simulink model "Drone_Failure"  (R2020a)
settings: Solver=VariableStepAuto  StartTime=0.0  StopTime=10.0  RelTol=1e-3
undefined symbols (not defined in the file): b, desired_gamma, desired_phi, desired_theta, desired_X, desired_Y, desired_Z, g, Ir, Ixx, Iyy, Izz, k, l, m
libraries: simulink x3
settings Model: Creator=prans  LastModifiedBy=prans
settings SolverCC: MaxConsecutiveMinStep=5

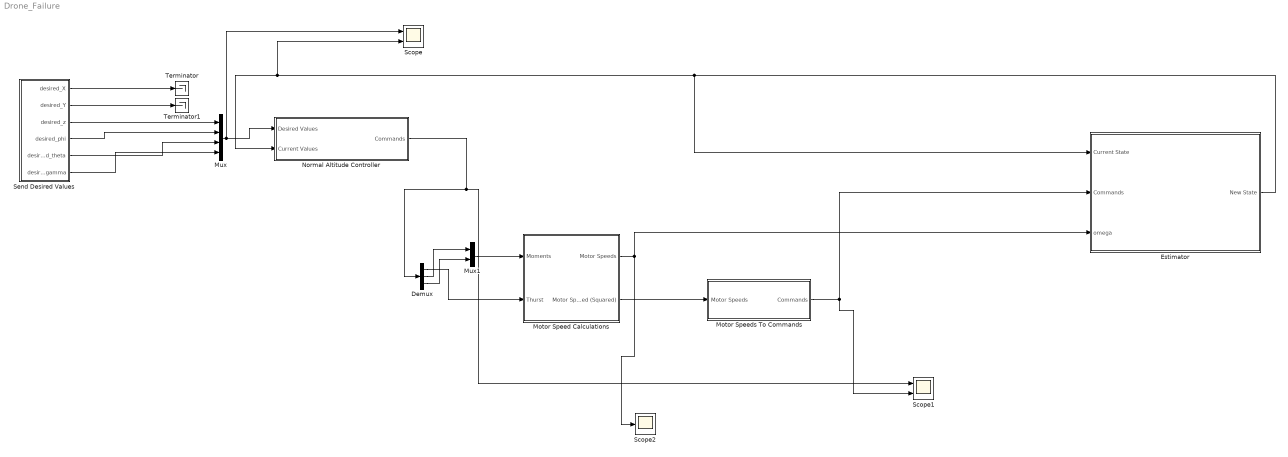
== system Drone_Failure ==
  Demux : Demux  Outputs=3
  Estimator : Subsystem
  Motor Speed Calculations : Subsystem
  Motor Speeds To Commands : Subsystem
  Mux : Mux
  Mux1 : Mux  Inputs=2
  Normal Altitude Controller : Subsystem
  Scope : Scope  NumInputPorts=2
  Scope1 : Scope  NumInputPorts=2
  Scope2 : Scope
  Send Desired Values : Subsystem
  Terminator : Terminator
  Terminator1 : Terminator
  wires:
  Send Desired Values/6(desired_gamma) -> Mux/4
  Send Desired Values/1(desired_X) -> Terminator/1
  Motor Speeds To Commands/1(Commands) -> Scope1/2, Estimator/2(Commands)
  Mux1/1 -> Motor Speed Calculations/1(Moments)
  Normal Altitude Controller/1(Commands) -> Scope1/1, Demux/1
  Motor Speed Calculations/1(Motor Speeds) -> Scope2/1, Estimator/3(omega)
  Send Desired Values/4(desired_phi) -> Mux/2
  Send Desired Values/5(desired_theta) -> Mux/3
  Demux/2 -> Mux1/1
  Send Desired Values/3(desired_z) -> Mux/1
  Send Desired Values/2(desired_Y) -> Terminator1/1
  Estimator/1(New State) -> Estimator/1(Current State), Scope/2, Normal Altitude Controller/2(Current Values)
  Demux/1 -> Motor Speed Calculations/2(Thurst)
  Mux/1 -> Scope/1, Normal Altitude Controller/1("Desired Values ")
  Demux/3 -> Mux1/2
  Motor Speed Calculations/2(Motor Speed (Squared)) -> Motor Speeds To Commands/1(Motor Speeds)

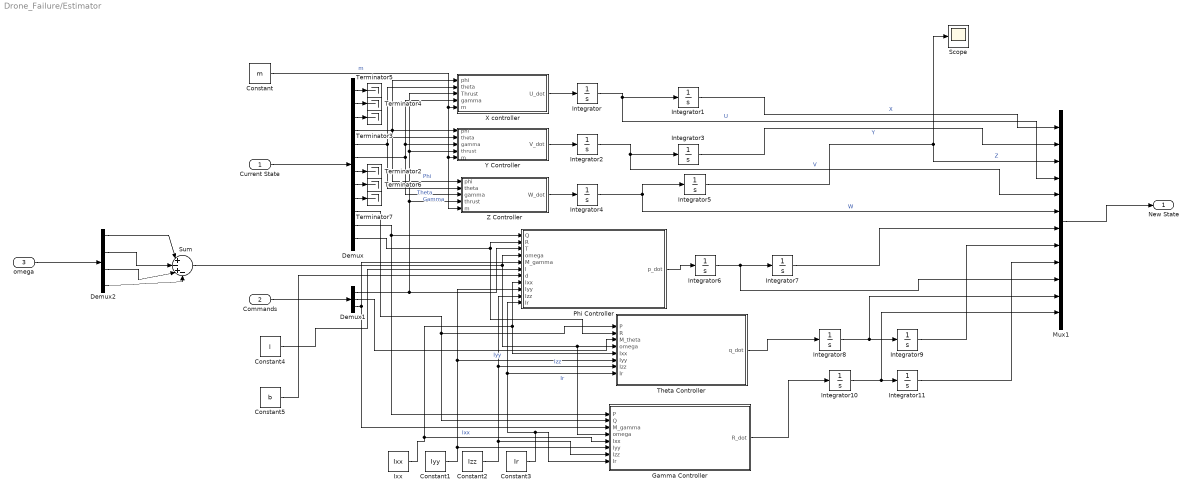
== system Drone_Failure/Estimator ==
  Current State : Inport
  Commands : Inport  Port=2
  omega : Inport  Port=3
  Constant : Constant  Value=m
  Constant1 : Constant  Value=Iyy
  Constant2 : Constant  Value=Izz
  Constant3 : Constant  Value=Ir
  Constant4 : Constant  Value=l
  Constant5 : Constant  Value=b
  Demux : Demux  Outputs=12
  Demux1 : Demux  Outputs=3
  Demux2 : Demux
  Gamma Controller : MATLAB Function  TreatAsAtomicUnit=on
  Integrator{,1..11} (12 alike) : Integrator
  Ixx : Constant  Value=Ixx
  Mux1 : Mux  Inputs=12
  Phi Controller : MATLAB Function  TreatAsAtomicUnit=on
  Scope : Scope
  Sum : Sum  Inputs=|+-+-
  Terminator{2..7} (6 alike) : Terminator
  Theta Controller : MATLAB Function  TreatAsAtomicUnit=on
  X controller : MATLAB Function  TreatAsAtomicUnit=on
  Y Controller : MATLAB Function  TreatAsAtomicUnit=on
  Z Controller : MATLAB Function  TreatAsAtomicUnit=on
  New State : Outport
  wires:
  Integrator8/1 -> Mux1/11, Integrator9/1
  Integrator6/1 -> Mux1/10, Integrator7/1
  Integrator9/1 -> Mux1/8
  Demux/11 -> Gamma Controller/1(P), Phi Controller/1(Q)
  Demux/9 -> Terminator7/1
  Demux/5 -> Y Controller/2(theta), X controller/2(theta), Z Controller/2(theta)  "Theta"
  Demux/2 -> Terminator4/1
  Demux/6 -> Y Controller/3(gamma), X controller/4(gamma), Z Controller/3(gamma)  "Gamma"
  Integrator1/1 -> Mux1/1  "X"
  Z Controller/1(W_dot) -> Integrator4/1
  Demux/3 -> Terminator3/1
  Gamma Controller/1(R_dot) -> Integrator10/1
  Current State/1 -> Demux/1
  Demux/10 -> Gamma Controller/2(Q), Theta Controller/1(P)
  Demux/8 -> Terminator6/1
  Demux/4 -> Z Controller/1(phi), Y Controller/1(phi), X controller/1(phi)  "Phi"
  Demux/7 -> Terminator2/1
  Integrator7/1 -> Mux1/7
  Demux/1 -> Terminator5/1
  Integrator11/1 -> Mux1/9
  Mux1/1 -> New State/1
  X controller/1(U_dot) -> Integrator/1
  Theta Controller/1(q_dot) -> Integrator8/1
  Integrator2/1 -> Integrator3/1, Mux1/5  "V"
  Phi Controller/1(p_dot) -> Integrator6/1
  Commands/1 -> Demux1/1
  Integrator3/1 -> Mux1/2  "Y"
  Y Controller/1(V_dot) -> Integrator2/1
  Demux/12 -> Theta Controller/2(R), Phi Controller/2(R)
  Integrator10/1 -> Mux1/12, Integrator11/1
  Integrator5/1 -> Scope/1, Mux1/3  "Z"
  Integrator/1 -> Integrator1/1, Mux1/4  "U"
  Integrator4/1 -> Integrator5/1, Mux1/6  "W"
  Ixx/1 -> Phi Controller/8(Ixx), Theta Controller/5(Ixx), Gamma Controller/5(Ixx)  "Ixx"
  Constant1/1 -> Phi Controller/9(Iyy), Theta Controller/6(Iyy), Gamma Controller/6(Iyy)  "Iyy"
  Constant2/1 -> Phi Controller/10(Izz), Theta Controller/7(Izz), Gamma Controller/7(Izz)  "Izz"
  Constant3/1 -> Phi Controller/11(Ir), Theta Controller/8(Ir), Gamma Controller/8(Ir)  "Ir"
  Constant/1 -> Z Controller/5(m), Y Controller/5(m), X controller/5(m)  "m"
  omega/1 -> Demux2/1
  Demux2/1 -> Sum/1
  Demux2/2 -> Sum/2
  Demux2/3 -> Sum/3
  Demux2/4 -> Sum/4
  Sum/1 -> Gamma Controller/4(omega), Theta Controller/4(omega), Phi Controller/4(omega)
  Demux1/1 -> X controller/3(Thrust), Y Controller/4(thrust), Z Controller/4(thrust), Phi Controller/3(T)
  Demux1/3 -> Phi Controller/5(M_gamma), Gamma Controller/3(M_gamma)
  Constant4/1 -> Phi Controller/6(l)
  Constant5/1 -> Phi Controller/7(d)
  Demux1/2 -> Theta Controller/3(M_theta)

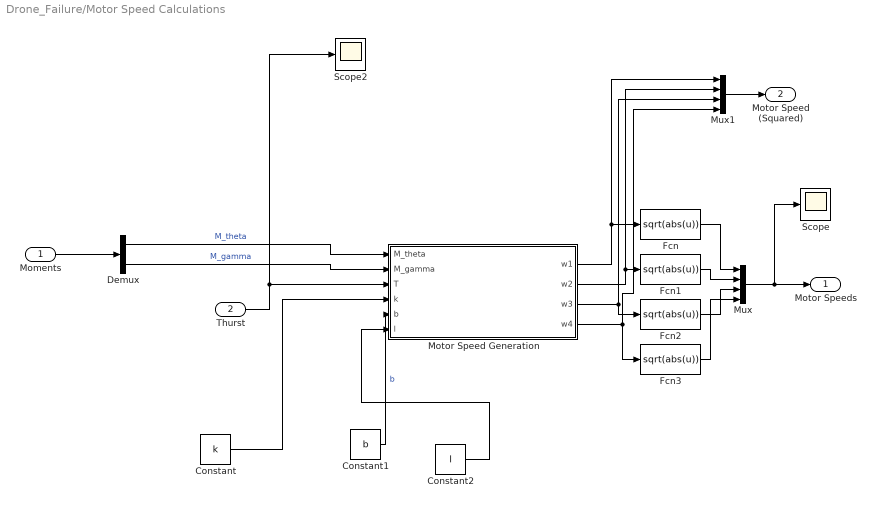
== system Drone_Failure/Motor Speed Calculations ==
  Moments : Inport
  Thurst : Inport  Port=2
  Constant : Constant  Value=k
  Constant1 : Constant  Value=b
  Constant2 : Constant  Value=l
  Demux : Demux  Outputs=2
  Fcn{,1..3} (4 alike) : Fcn  Expr=sqrt(abs(u))
  Motor Speed Generation : MATLAB Function  TreatAsAtomicUnit=on
  Mux : Mux
  Mux1 : Mux
  Scope : Scope
  Scope2 : Scope
  Motor Speeds : Outport
  Motor Speed (Squared) : Outport  Port=2
  wires:
  Motor Speed Generation/4(w4) -> Fcn3/1, Mux1/4
  Motor Speed Generation/2(w2) -> Mux1/2, Fcn1/1
  Thurst/1 -> Scope2/1, Motor Speed Generation/3(T)
  Motor Speed Generation/1(w1) -> Mux1/1, Fcn/1
  Motor Speed Generation/3(w3) -> Fcn2/1, Mux1/3
  Moments/1 -> Demux/1
  Mux/1 -> Scope/1, Motor Speeds/1
  Constant/1 -> Motor Speed Generation/4(k)
  Constant1/1 -> Motor Speed Generation/5(b)  "b"
  Demux/1 -> Motor Speed Generation/1(M_theta)  "M_theta"
  Demux/2 -> Motor Speed Generation/2(M_gamma)  "M_gamma"
  Constant2/1 -> Motor Speed Generation/6(l)
  Fcn/1 -> Mux/1
  Fcn1/1 -> Mux/2
  Fcn2/1 -> Mux/3
  Fcn3/1 -> Mux/4
  Mux1/1 -> Motor Speed (Squared)/1

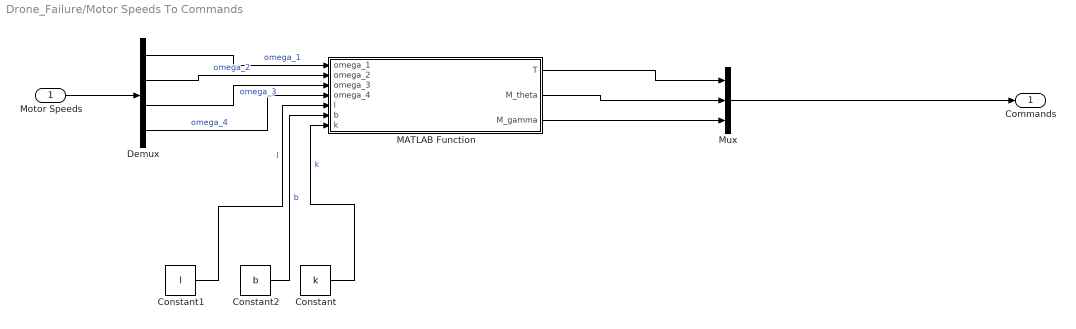
== system Drone_Failure/Motor Speeds To Commands ==
  Motor Speeds : Inport
  Constant : Constant  Value=k
  Constant1 : Constant  Value=l
  Constant2 : Constant  Value=b
  Demux : Demux
  MATLAB Function : MATLAB Function  TreatAsAtomicUnit=on
  Mux : Mux  Inputs=3
  Commands : Outport
  wires:
  Constant2/1 -> MATLAB Function/6(b)  "b"
  Demux/2 -> MATLAB Function/2(omega_2)  "omega_2"
  Constant/1 -> MATLAB Function/7(k)  "k"
  MATLAB Function/3(M_gamma) -> Mux/3
  Constant1/1 -> MATLAB Function/5(l)  "l"
  MATLAB Function/2(M_theta) -> Mux/2
  MATLAB Function/1(T) -> Mux/1
  Demux/3 -> MATLAB Function/3(omega_3)  "omega_3"
  Demux/1 -> MATLAB Function/1(omega_1)  "omega_1"
  Demux/4 -> MATLAB Function/4(omega_4)  "omega_4"
  Mux/1 -> Commands/1
  Motor Speeds/1 -> Demux/1

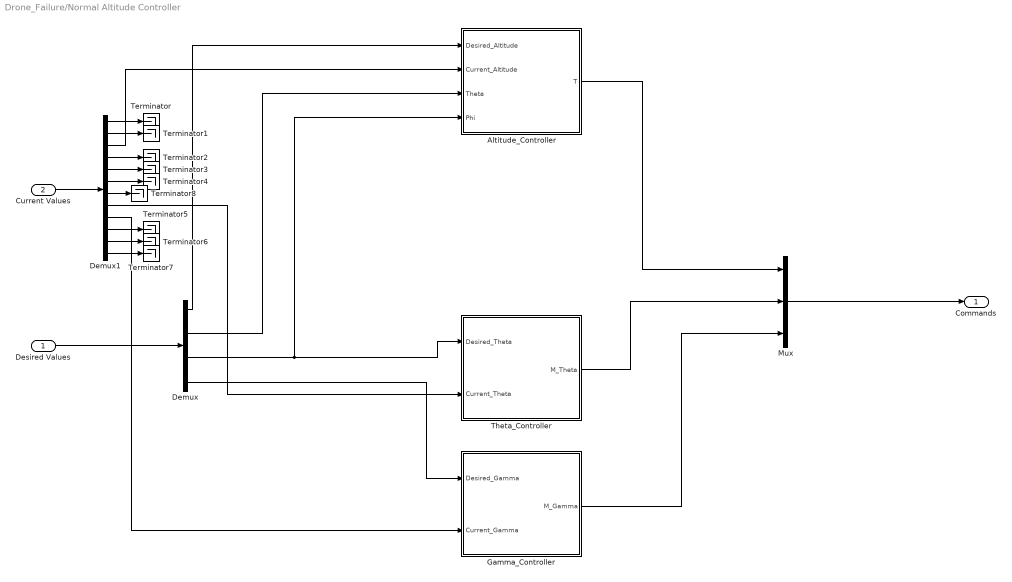
== system Drone_Failure/Normal Altitude Controller ==
  "Desired Values " : Inport
  Current Values : Inport  Port=2
  Altitude_Controller : Subsystem
  Demux : Demux
  Demux1 : Demux  Outputs=12
  Gamma_Controller : Subsystem
  Mux : Mux  Inputs=3
  Terminator{,1..8} (9 alike) : Terminator
  Theta_Controller : Subsystem
  Commands : Outport
  wires:
  Demux/1 -> Altitude_Controller/1(Desired_Altitude)
  "Desired Values "/1 -> Demux/1
  Current Values/1 -> Demux1/1
  Demux/3 -> Altitude_Controller/4(Phi), Theta_Controller/1(Desired_Theta)
  Demux/4 -> Gamma_Controller/1(Desired_Gamma)
  Theta_Controller/1(M_Theta) -> Mux/2
  Altitude_Controller/1(T) -> Mux/1
  Mux/1 -> Commands/1
  Demux1/3 -> Altitude_Controller/2(Current_Altitude)
  Gamma_Controller/1(M_Gamma) -> Mux/3
  Demux/2 -> Altitude_Controller/3(Theta)
  Demux1/1 -> Terminator/1
  Demux1/2 -> Terminator1/1
  Demux1/8 -> Theta_Controller/2(Current_Theta)
  Demux1/9 -> Gamma_Controller/2(Current_Gamma)
  Demux1/10 -> Terminator5/1
  Demux1/11 -> Terminator6/1
  Demux1/12 -> Terminator7/1
  Demux1/4 -> Terminator2/1
  Demux1/5 -> Terminator3/1
  Demux1/6 -> Terminator4/1
  Demux1/7 -> Terminator8/1

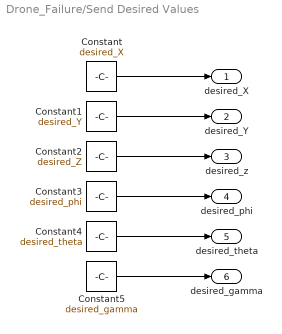
== system Drone_Failure/Send Desired Values ==
  Constant : Constant  Value=desired_X
  Constant1 : Constant  Value=desired_Y
  Constant2 : Constant  Value=desired_Z
  Constant3 : Constant  Value=desired_phi
  Constant4 : Constant  Value=desired_theta
  Constant5 : Constant  Value=desired_gamma
  desired_X : Outport
  desired_Y : Outport  Port=2
  desired_z : Outport  Port=3
  desired_phi : Outport  Port=4
  desired_theta : Outport  Port=5
  desired_gamma : Outport  Port=6
  wires:
  Constant/1 -> desired_X/1
  Constant1/1 -> desired_Y/1
  Constant2/1 -> desired_z/1
  Constant3/1 -> desired_phi/1
  Constant4/1 -> desired_theta/1
  Constant5/1 -> desired_gamma/1

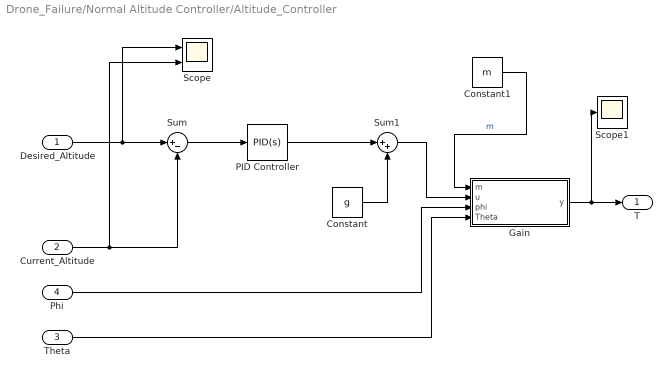
== system Drone_Failure/Normal Altitude Controller/Altitude_Controller ==
  Desired_Altitude : Inport
  Current_Altitude : Inport  Port=2
  Theta : Inport  Port=3
  Phi : Inport  Port=4
  Constant : Constant  Value=g
  Constant1 : Constant  Value=m
  Gain : MATLAB Function  TreatAsAtomicUnit=on
  PID Controller : simulink/Continuous/PID Controller  Controller=PID  Form=Parallel  TimeDomain=Continuous-time  UseExternalTs=off  SampleTime=-1  IntegratorMethod=Forward Euler  FilterMethod=Forward Euler  ControllerParametersSource=internal  P=1  I=1  D=0  UseFilter=on  N=54.5397025421619  TunerSelectOption=Transfer Function Based (PID Tuner App)  InitialConditionSource=internal  InitialConditionForIntegrator=0  InitialConditionForFilter=0  DifferentiatorICPrevScaledInput=0  ExternalReset=none  TrackingMode=off  Kt=1  LimitOutput=off  UpperSaturationLimit=inf  LowerSaturationLimit=-inf  LinearizeAsGain=on  AntiWindupMode=none  Kb=1  POutMin=[]  POutMax=[]  IOutMin=[]  IOutMax=[]  DOutMin=[]  DOutMax=[]  NOutMin=[]  NOutMax=[]  SumOutMin=[]  SumOutMax=[]  SaturationOutMin=[]  SaturationOutMax=[]  PParamMin=[]  PParamMax=[]  IParamMin=[]  IParamMax=[]  DParamMin=[]  DParamMax=[]  NParamMin=[]  NParamMax=[]  KbParamMin=[]  KbParamMax=[]  KtParamMin=[]  KtParamMax=[]  KbOutMin=[]  KbOutMax=[]  KtOutMin=[]  KtOutMax=[]  IntegratorOutMin=[]  IntegratorOutMax=[]  FilterOutMin=[]  FilterOutMax=[]  SumI1OutMin=[]  SumI1OutMax=[]  SumI2OutMin=[]  SumI2OutMax=[]  SumI3OutMin=[]  SumI3OutMax=[]  SumI4OutMin=[]  SumI4OutMax=[]  SumDOutMin=[]  SumDOutMax=[]  DifferentiatorOutMin=[]  DifferentiatorOutMax=[]  FilterDiffOutCoefMin=[]  FilterDiffOutCoefMax=[]  ReciprocalOutMin=[]  ReciprocalOutMax=[]  SumDenOutMin=[]  SumDenOutMax=[]  SumNumOutMin=[]  SumNumOutMax=[]  DivideOutMin=[]  DivideOutMax=[]  UdiffTsProdOutMin=[]  UdiffTsProdOutMax=[]  NTsProdOutMin=[]  NTsProdOutMax=[]  UintegralTsProdOutMin=[]  UintegralTsProdOutMax=[]  UngainTsProdOutMin=[]  UngainTsProdOutMax=[]  IntegratorContinuousStateAttributes=''  IntegratorStateMustResolveToSignalObject=off  IntegratorRTWStateStorageClass=Auto  FilterContinuousStateAttributes=''  FilterStateMustResolveToSignalObject=off  FilterRTWStateStorageClass=Auto  ParallelPVariant=InternalParameters  IdealPVariant=Disabled  IVariant=InternalParameters  DVariant=InternalParameters  IntegratorVariant=Continuous  SatVariant=Disabled  AWVariant=Passthrough  PCopyVariant=Disabled  TRVariant=Disabled  FdbkBlocksVariant=Forward  IdealPFdbkVariant=Disabled  SatFdbkVariant=Disabled  DerivativeFilterVariant=ContFilter  NVariant=InternalParameters  NCopyVariant=Disabled  FilterICVariant=InternalICsFilter  IntegratorICVariant=InternalICs  ExternalResetVariant=Disabled  TRSumVariant=Passthrough  SumFdbkVariant=Disabled  SumVariant=Sum_PID  TsampFilterVariant=InternalTs  TsampNgainVariant=Passthrough  TsampIntegralVariant=Passthrough
  Scope : Scope  NumInputPorts=2
  Scope1 : Scope
  Sum : Sum  Inputs=|+-
  Sum1 : Sum  Inputs=|++
  T : Outport
  wires:
  Sum/1 -> PID Controller/1
  PID Controller/1 -> Sum1/1
  Current_Altitude/1 -> Scope/2, Sum/2
  Desired_Altitude/1 -> Scope/1, Sum/1
  Gain/1(y) -> Scope1/1, T/1
  Sum1/1 -> Gain/2(u)
  Constant/1 -> Sum1/2
  Phi/1 -> Gain/3(phi)
  Theta/1 -> Gain/4(Theta)
  Constant1/1 -> Gain/1(m)  "m"

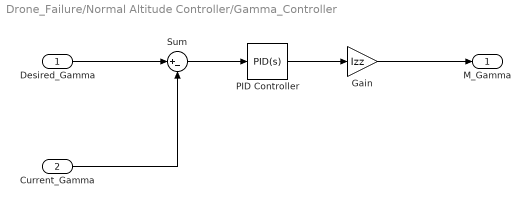
== system Drone_Failure/Normal Altitude Controller/Gamma_Controller ==
  Desired_Gamma : Inport
  Current_Gamma : Inport  Port=2
  Gain : Gain  Gain=Izz
  PID Controller : simulink/Continuous/PID Controller  Controller=PID  Form=Parallel  TimeDomain=Continuous-time  UseExternalTs=off  SampleTime=-1  IntegratorMethod=Forward Euler  FilterMethod=Forward Euler  ControllerParametersSource=internal  P=1  I=1  D=0  UseFilter=on  N=100  TunerSelectOption=Transfer Function Based (PID Tuner App)  InitialConditionSource=internal  InitialConditionForIntegrator=0  InitialConditionForFilter=0  DifferentiatorICPrevScaledInput=0  ExternalReset=none  TrackingMode=off  Kt=1  LimitOutput=off  UpperSaturationLimit=inf  LowerSaturationLimit=-inf  LinearizeAsGain=on  AntiWindupMode=none  Kb=1  POutMin=[]  POutMax=[]  IOutMin=[]  IOutMax=[]  DOutMin=[]  DOutMax=[]  NOutMin=[]  NOutMax=[]  SumOutMin=[]  SumOutMax=[]  SaturationOutMin=[]  SaturationOutMax=[]  PParamMin=[]  PParamMax=[]  IParamMin=[]  IParamMax=[]  DParamMin=[]  DParamMax=[]  NParamMin=[]  NParamMax=[]  KbParamMin=[]  KbParamMax=[]  KtParamMin=[]  KtParamMax=[]  KbOutMin=[]  KbOutMax=[]  KtOutMin=[]  KtOutMax=[]  IntegratorOutMin=[]  IntegratorOutMax=[]  FilterOutMin=[]  FilterOutMax=[]  SumI1OutMin=[]  SumI1OutMax=[]  SumI2OutMin=[]  SumI2OutMax=[]  SumI3OutMin=[]  SumI3OutMax=[]  SumI4OutMin=[]  SumI4OutMax=[]  SumDOutMin=[]  SumDOutMax=[]  DifferentiatorOutMin=[]  DifferentiatorOutMax=[]  FilterDiffOutCoefMin=[]  FilterDiffOutCoefMax=[]  ReciprocalOutMin=[]  ReciprocalOutMax=[]  SumDenOutMin=[]  SumDenOutMax=[]  SumNumOutMin=[]  SumNumOutMax=[]  DivideOutMin=[]  DivideOutMax=[]  UdiffTsProdOutMin=[]  UdiffTsProdOutMax=[]  NTsProdOutMin=[]  NTsProdOutMax=[]  UintegralTsProdOutMin=[]  UintegralTsProdOutMax=[]  UngainTsProdOutMin=[]  UngainTsProdOutMax=[]  IntegratorContinuousStateAttributes=''  IntegratorStateMustResolveToSignalObject=off  IntegratorRTWStateStorageClass=Auto  FilterContinuousStateAttributes=''  FilterStateMustResolveToSignalObject=off  FilterRTWStateStorageClass=Auto  ParallelPVariant=InternalParameters  IdealPVariant=Disabled  IVariant=InternalParameters  DVariant=InternalParameters  IntegratorVariant=Continuous  SatVariant=Disabled  AWVariant=Passthrough  PCopyVariant=Disabled  TRVariant=Disabled  FdbkBlocksVariant=Forward  IdealPFdbkVariant=Disabled  SatFdbkVariant=Disabled  DerivativeFilterVariant=ContFilter  NVariant=InternalParameters  NCopyVariant=Disabled  FilterICVariant=InternalICsFilter  IntegratorICVariant=InternalICs  ExternalResetVariant=Disabled  TRSumVariant=Passthrough  SumFdbkVariant=Disabled  SumVariant=Sum_PID  TsampFilterVariant=InternalTs  TsampNgainVariant=Passthrough  TsampIntegralVariant=Passthrough
  Sum : Sum  Inputs=|+-
  M_Gamma : Outport
  wires:
  Sum/1 -> PID Controller/1
  PID Controller/1 -> Gain/1
  Current_Gamma/1 -> Sum/2
  Desired_Gamma/1 -> Sum/1
  Gain/1 -> M_Gamma/1

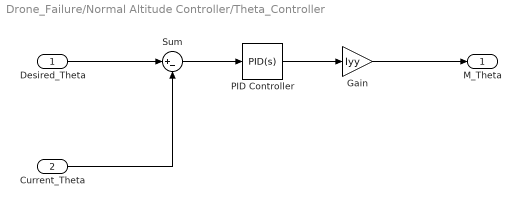
== system Drone_Failure/Normal Altitude Controller/Theta_Controller ==
  Desired_Theta : Inport
  Current_Theta : Inport  Port=2
  Gain : Gain  Gain=Iyy
  PID Controller : simulink/Continuous/PID Controller  Controller=PID  Form=Parallel  TimeDomain=Continuous-time  UseExternalTs=off  SampleTime=-1  IntegratorMethod=Forward Euler  FilterMethod=Forward Euler  ControllerParametersSource=internal  P=1  I=1  D=0  UseFilter=on  N=100  TunerSelectOption=Transfer Function Based (PID Tuner App)  InitialConditionSource=internal  InitialConditionForIntegrator=0  InitialConditionForFilter=0  DifferentiatorICPrevScaledInput=0  ExternalReset=none  TrackingMode=off  Kt=1  LimitOutput=off  UpperSaturationLimit=inf  LowerSaturationLimit=-inf  LinearizeAsGain=on  AntiWindupMode=none  Kb=1  POutMin=[]  POutMax=[]  IOutMin=[]  IOutMax=[]  DOutMin=[]  DOutMax=[]  NOutMin=[]  NOutMax=[]  SumOutMin=[]  SumOutMax=[]  SaturationOutMin=[]  SaturationOutMax=[]  PParamMin=[]  PParamMax=[]  IParamMin=[]  IParamMax=[]  DParamMin=[]  DParamMax=[]  NParamMin=[]  NParamMax=[]  KbParamMin=[]  KbParamMax=[]  KtParamMin=[]  KtParamMax=[]  KbOutMin=[]  KbOutMax=[]  KtOutMin=[]  KtOutMax=[]  IntegratorOutMin=[]  IntegratorOutMax=[]  FilterOutMin=[]  FilterOutMax=[]  SumI1OutMin=[]  SumI1OutMax=[]  SumI2OutMin=[]  SumI2OutMax=[]  SumI3OutMin=[]  SumI3OutMax=[]  SumI4OutMin=[]  SumI4OutMax=[]  SumDOutMin=[]  SumDOutMax=[]  DifferentiatorOutMin=[]  DifferentiatorOutMax=[]  FilterDiffOutCoefMin=[]  FilterDiffOutCoefMax=[]  ReciprocalOutMin=[]  ReciprocalOutMax=[]  SumDenOutMin=[]  SumDenOutMax=[]  SumNumOutMin=[]  SumNumOutMax=[]  DivideOutMin=[]  DivideOutMax=[]  UdiffTsProdOutMin=[]  UdiffTsProdOutMax=[]  NTsProdOutMin=[]  NTsProdOutMax=[]  UintegralTsProdOutMin=[]  UintegralTsProdOutMax=[]  UngainTsProdOutMin=[]  UngainTsProdOutMax=[]  IntegratorContinuousStateAttributes=''  IntegratorStateMustResolveToSignalObject=off  IntegratorRTWStateStorageClass=Auto  FilterContinuousStateAttributes=''  FilterStateMustResolveToSignalObject=off  FilterRTWStateStorageClass=Auto  ParallelPVariant=InternalParameters  IdealPVariant=Disabled  IVariant=InternalParameters  DVariant=InternalParameters  IntegratorVariant=Continuous  SatVariant=Disabled  AWVariant=Passthrough  PCopyVariant=Disabled  TRVariant=Disabled  FdbkBlocksVariant=Forward  IdealPFdbkVariant=Disabled  SatFdbkVariant=Disabled  DerivativeFilterVariant=ContFilter  NVariant=InternalParameters  NCopyVariant=Disabled  FilterICVariant=InternalICsFilter  IntegratorICVariant=InternalICs  ExternalResetVariant=Disabled  TRSumVariant=Passthrough  SumFdbkVariant=Disabled  SumVariant=Sum_PID  TsampFilterVariant=InternalTs  TsampNgainVariant=Passthrough  TsampIntegralVariant=Passthrough
  Sum : Sum  Inputs=|+-
  M_Theta : Outport
  wires:
  Sum/1 -> PID Controller/1
  PID Controller/1 -> Gain/1
  Current_Theta/1 -> Sum/2
  Desired_Theta/1 -> Sum/1
  Gain/1 -> M_Theta/1

== matlab function Drone_Failure/Motor Speed Calculations/Motor Speed Generation ==
  data: M_theta input; M_gamma input; w1 output; w2 output; T input; w3 output; w4 output; k input; b input; l input
function [w1,w2,w3,w4] = fcn(M_theta, M_gamma, T,k, b, l)
w1 = T/(4*k) - M_theta/(2*k*l) - M_gamma/(4*b);
% w2 = T/(4*k) - M_phi/(2*k*l) + M_gamma/(4*b);
w2 = 0;
w3 = T/(4*k) + M_theta/(2*k*l) - M_gamma/(4*b);
w4 = T/(4*k) + M_gamma/(4*b);

== matlab function Drone_Failure/Motor Speeds To Commands/MATLAB Function ==
  data: omega_1 input; T output; omega_2 input; omega_3 input; omega_4 input; l input; b input; k input; M_theta output; M_gamma output
function [T,M_theta,M_gamma] = fcn(omega_1, omega_2, omega_3, omega_4, l, b, k)

% omega_1 = omega_1^2;
% omega_2 = omega_2^2;
% omega_3 = omega_3^2;
% omega_4 = omega_4^2;

T = k*(omega_1+ omega_2 + omega_3 + omega_4);
% M_phi = k*l*omega_2 - k*l*omega_4;
M_theta = -k*l*omega_1 + k*l*omega_3;
M_gamma = b*(-omega_1 - omega_3 + omega_4);

== matlab function Drone_Failure/Estimator/X controller ==
  data: phi input; theta input; Thrust input; U_dot output; gamma input; m input
function U_dot = fcn(phi, theta, Thrust, gamma, m)

U_dot = (sin(phi)*sin(gamma) + cos(phi)*cos(gamma)*sin(theta))*Thrust/m;

== matlab function Drone_Failure/Normal Altitude Controller/Altitude_Controller/Gain ==
  data: m input; u input; y output; phi input; Theta input
function y = fcn(m, u, phi, Theta)

y = cos(phi)*cos(Theta)*m*u;

== matlab function Drone_Failure/Estimator/Y Controller ==
  data: phi input; theta input; V_dot output; gamma input; thrust input; m input
function V_dot = fcn(phi, theta, gamma, thrust, m)

V_dot = (-sin(phi)*cos(gamma) + cos(phi)*sin(theta)*sin(gamma))*thrust/m;

== matlab function Drone_Failure/Estimator/Phi Controller ==
  data: Q input; R input; p_dot output; T input; omega input; M_gamma input; l input; d input; Ixx input; Iyy input; Izz input; Ir input
function p_dot = fcn(Q, R,T, omega, M_gamma,l,d, Ixx, Iyy, Izz, Ir)

p_dot = (Ixx - Iyy)/(Izz)*Q*R - (Ir/Ixx)*Q*omega + 0.5*l*(T - (M_gamma/d))/Ixx;

== matlab function Drone_Failure/Estimator/Theta Controller ==
  data: P input; R input; q_dot output; M_theta input; omega input; Ixx input; Iyy input; Izz input; Ir input
function q_dot = fcn(P, R, M_theta, omega, Ixx, Iyy, Izz, Ir)

q_dot = ((Izz - Ixx)/Iyy)*P*R - Ir/Iyy*P*omega + M_theta/Iyy;

== matlab function Drone_Failure/Estimator/Gamma Controller ==
  data: P input; Q input; R_dot output; M_gamma input; omega input; Ixx input; Iyy input; Izz input; Ir input
function R_dot = fcn(P, Q, M_gamma, omega, Ixx, Iyy, Izz, Ir)

R_dot = ((Ixx-Iyy)/Izz)*P*Q + M_gamma/Izz;

== matlab function Drone_Failure/Estimator/Z Controller ==
  data: phi input; theta input; W_dot output; gamma input; thrust input; m input
function W_dot = fcn(phi, theta, gamma, thrust, m)

W_dot = -9.81 + (cos(phi)*cos(theta))*thrust/m;
